simulink model "trackRobotStates"  (R2023a)
settings: Solver=ode3  StartTime=0.0  StopTime=inf  FixedStep=sampleTime  RelTol=1e-3
PreLoadFcn:
  | currentPath = pwd;
  | rootLocation = fileparts(currentPath);
  | if ~exist('JacoComm.m', 'file')
  |     addpath(fullfile(rootLocation, 'Source'));
  | end
PostLoadFcn:
  | q_home = [4.806;2.924;1.004;4.204;1.445;1.323];
  | sampleTime = 0.1;
InitFcn:
  | cd(fullfile(rootLocation, 'JACO2SDK'));
StartFcn:
  | cd(currentPath);
model workspace (MAT data in the model file):
  sampleTime = 0.1
libraries: aerolibanimutils x1
settings Model: Creator=csantacr  LastModifiedBy=saswt
settings SolverCC: AlgebraicLoopSolver=TrustRegion
settings DataIOCC: ReturnWorkspaceOutputs=off
settings OptimizationCC: ZeroExternalMemoryAtStartup=off  ZeroInternalMemoryAtStartup=off
settings DebuggingCC: UnconnectedInputMsg=warning  UnconnectedOutputMsg=warning  UnconnectedLineMsg=warning  ArithmeticOperatorsInVariantConditions=warning
settings ModelReferenceCC: EnableRefExpFcnMdlSchedulingChecks=on
settings SFSimCC: SimUseLocalCustomCode=off  CustomCodeUndefinedFunction=UseInterfaceOnly  SimTargetLang=C++
settings RTWCC: RTWUseLocalCustomCode=off  RTWUseSimCustomCode=on  Toolchain=Microsoft Visual C++ 2015 v14.0 | nmake (64-bit Windows)  TargetLang=C++
settings CodeAppCC: StateflowObjectComments=on
settings GRTTargetCC: TargetLangStandard=C++03 (ISO)  CodeInterfacePackaging=C++ class

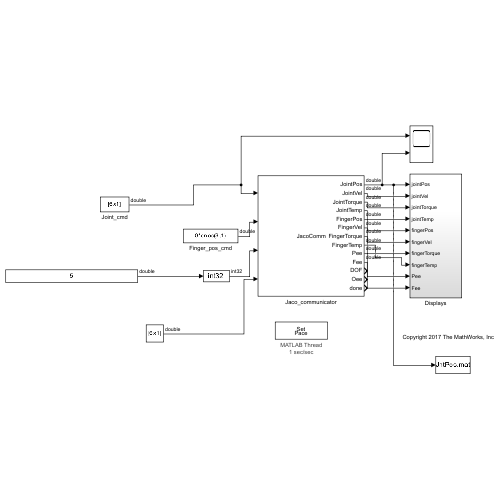
[thumbnail: Simulink's stored preview of the top-level diagram]
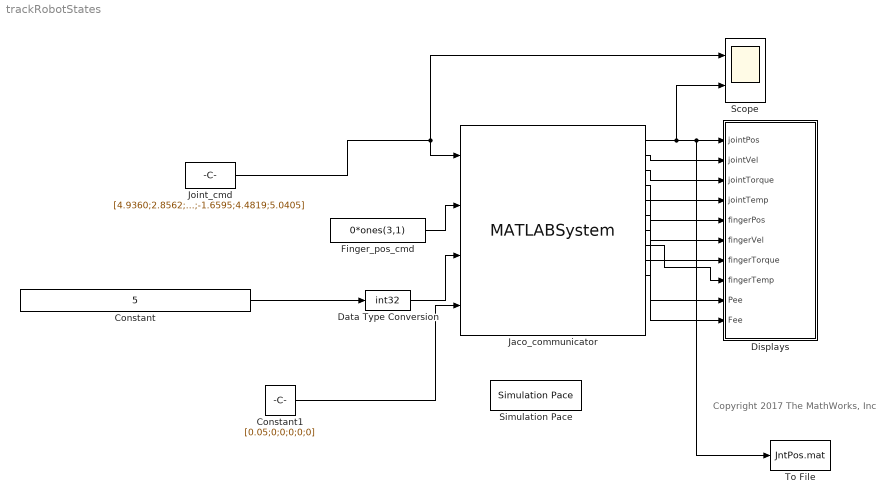
== system trackRobotStates ==
  note: Copyright 2017 The MathWorks, Inc
  Constant : Constant  Value=5
  Constant1 : Constant  Value=[0.05;0;0;0;0;0]
  Data Type Conversion : DataTypeConversion  OutDataTypeStr=int32  SaturateOnIntegerOverflow=off  RndMeth=Floor
  Displays : Subsystem
  Finger_pos_cmd : Constant  Value=0*ones(3,1)
  Jaco_communicator : MATLABSystem  System=JacoComm  ControlMode=Position  CalibrateFingersAtStartup=off  GoToHomeAtStartup=off  SimulateUsing=Interpreted execution
      mask Type: JacoComm
      mask Display:
      | disp('JacoComm');
      | port_label('output',1,'JointPos');
      | port_label('output',2,'JointVel');
      | port_label('output',3,'JointTorque');
      | port_label('output',4,'JointTemp');
      | port_label('output',5,'FingerPos');
      | port_label('output',6,'FingerVel');
      | port_label('output',7,'FingerTorque');
      | port_label('output',8,'FingerTemp');
      | port_label('output',9,'Pee');
      | port_label('output',10,'Fee');
      | port_label('output',11,'DOF');
      | port_label('output',12,'Oee');
      | port_label('output',13,'done');
  Joint_cmd : Constant  Value=[4.9360;2.8562;0.7641;-1.6595;4.4819;5.0405]  SampleTime=sampleTime
  Scope : Scope  NumInputPorts=2
  Simulation Pace : aerolibanimutils/Simulation Pace  SimulationPace=1  SleepMode=MATLAB Thread  OutputPaceError=off  SampleTime=sampleTime
  To File : ToFile  Filename=JntPos.mat
  wires:
  Jaco_communicator/1 -> Scope/2, To File/1, Displays/1(jointPos)
  Joint_cmd/1 -> Jaco_communicator/1, Scope/1
  Finger_pos_cmd/1 -> Jaco_communicator/2
  Constant/1 -> Data Type Conversion/1
  Jaco_communicator/2 -> Displays/2(jointVel)
  Jaco_communicator/3 -> Displays/3(jointTorque)
  Jaco_communicator/4 -> Displays/4(jointTemp)
  Jaco_communicator/5 -> Displays/5(fingerPos)
  Jaco_communicator/6 -> Displays/6(fingerVel)
  Jaco_communicator/7 -> Displays/7(fingerTorque)
  Jaco_communicator/8 -> Displays/8(fingerTemp)
  Jaco_communicator/9 -> Displays/9(Pee)
  Jaco_communicator/10 -> Displays/10(Fee)
  Data Type Conversion/1 -> Jaco_communicator/3
  Constant1/1 -> Jaco_communicator/4

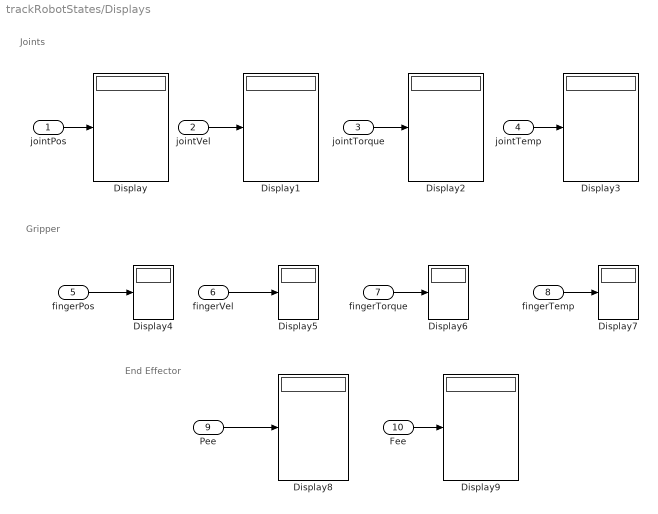
== system trackRobotStates/Displays ==
  note: End Effector
  note: Gripper
  note: Joints
  jointPos : Inport
  jointVel : Inport  Port=2
  jointTorque : Inport  Port=3
  jointTemp : Inport  Port=4
  fingerPos : Inport  Port=5
  fingerVel : Inport  Port=6
  fingerTorque : Inport  Port=7
  fingerTemp : Inport  Port=8
  Pee : Inport  Port=9
  Fee : Inport  Port=10
  Display{,1..9} (10 alike) : Display
  wires:
  jointTemp/1 -> Display3/1
  fingerPos/1 -> Display4/1
  fingerVel/1 -> Display5/1
  fingerTorque/1 -> Display6/1
  jointVel/1 -> Display1/1
  jointTorque/1 -> Display2/1
  Fee/1 -> Display9/1
  Pee/1 -> Display8/1
  fingerTemp/1 -> Display7/1
  jointPos/1 -> Display/1
